simulink model "VCP_interface_STM32F429"  (R2022b)
settings: Solver=FixedStepDiscrete  StartTime=0.0  StopTime=inf  FixedStep=Ts  RelTol=1e-3
InitFcn:
  | datafields_per_usb_transfer = 16;
  | bytes_per_usb_transfer = 16*4;
  | Ts = 10e-3;
libraries: instrumentseriallib x3
settings Model: Creator=oliver.dieterle  LastModifiedBy=oliver.dieterle
settings SolverCC: AlgebraicLoopSolver=TrustRegion
settings DataIOCC: LimitDataPoints=on  SaveFormat=Array  ReturnWorkspaceOutputs=off
settings OptimizationCC: BlockReduction=off  BooleanDataType=off  LifeSpan=inf
settings DebuggingCC: SaveWithParameterizedLinksMsg=none  UnderspecifiedInitializationDetection=Classic  MergeDetectMultiDrivingBlocksExec=none  SignalResolutionControl=TryResolveAllWithWarning  UnconnectedInputMsg=warning  UnconnectedOutputMsg=warning  UnconnectedLineMsg=warning  SFUnexpectedBacktrackingDiag=warning  SFNoUnconditionalDefaultTransitionDiag=warning  SFExecutionAtInitializationDiag=none  SFMachineParentedDataDiag=warning  ArithmeticOperatorsInVariantConditions=warning
settings HardwareCC: ProdBitPerPointer=32  ProdBitPerSizeT=32  ProdBitPerPtrDiffT=32  ProdLargestAtomicFloat=None  ProdIntDivRoundTo=Undefined  ProdEndianess=Unspecified  ProdWordSize=32  ProdHWDeviceType=32-bit Generic  TargetUnknown=on
settings ModelReferenceCC: EnableRefExpFcnMdlSchedulingChecks=on  PropagateSignalLabelsOutOfModel=off
settings SFSimCC: SimUseLocalCustomCode=off  CustomCodeUndefinedFunction=UseInterfaceOnly
settings RTWCC: RTWUseLocalCustomCode=off
settings CodeAppCC: StateflowObjectComments=on
settings GRTTargetCC: TargetLangStandard=C89/C90 (ANSI)
settings ConfigComp: CovMetricSettings=dw  CovSaveCumulativeToWorkspaceVar=on  CovSaveSingleToWorkspaceVar=on  CovExternalEMLEnable=off  CovSFcnEnable=off

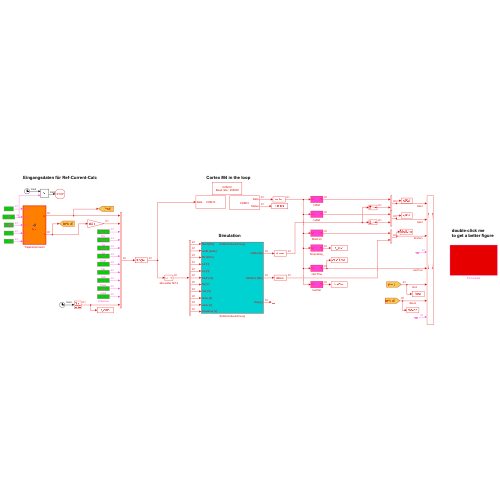
[thumbnail: Simulink's stored preview of the top-level diagram]
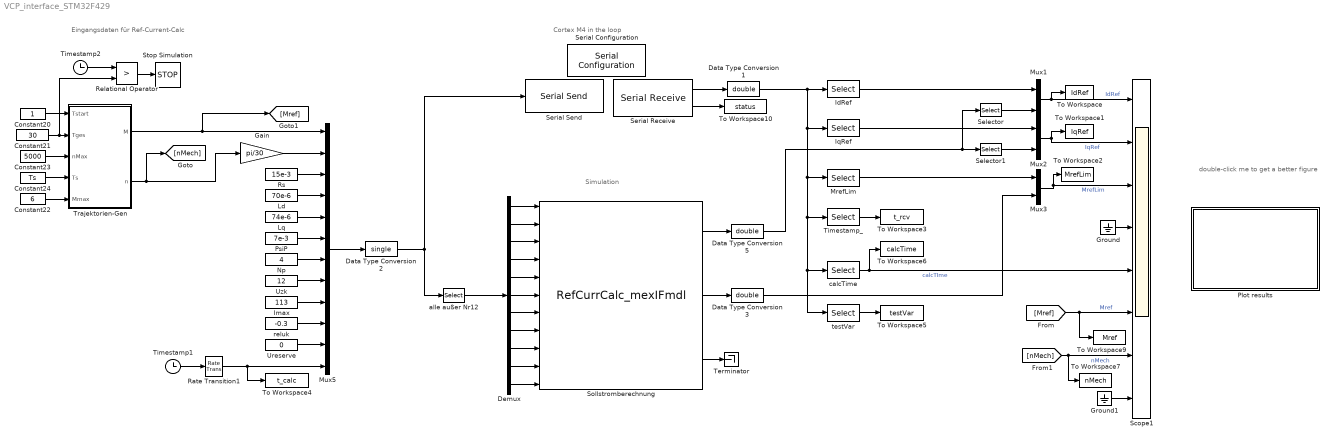
== system VCP_interface_STM32F429 ==
  note: Simulation
  note: Cortex M4 in the loop
  note: Eingangsdaten für Ref-Current-Calc
  note: double-click me
      | to get a better figure
  Constant20 : Constant
  Constant21 : Constant  Value=30
  Constant22 : Constant  Value=6
  Constant23 : Constant  Value=5000
  Constant24 : Constant  Value=Ts
  Data Type Conversion1 : DataTypeConversion  OutDataTypeStr=double  SaturateOnIntegerOverflow=off  RndMeth=Floor
  Data Type Conversion2 : DataTypeConversion  OutDataTypeStr=single  SaturateOnIntegerOverflow=off  RndMeth=Floor
  Data Type Conversion3 : DataTypeConversion  OutDataTypeStr=double  SaturateOnIntegerOverflow=off  RndMeth=Floor
  Data Type Conversion5 : DataTypeConversion  OutDataTypeStr=double  SaturateOnIntegerOverflow=off  RndMeth=Floor
  Demux : Demux  Outputs=11
  Gain : Gain  Gain=pi/30
  Ground : Ground
  Ground1 : Ground
  IdRef : Selector  InputPortWidth=datafields_per_usb_transfer  IndexOptions=Index vector (dialog)  Indices=1  OutputSizes=1
  Imax : Constant  Value=113
  IqRef : Selector  InputPortWidth=datafields_per_usb_transfer  IndexOptions=Index vector (dialog)  Indices=2  OutputSizes=1
  Ld : Constant  Value=70e-6
  Lq : Constant  Value=74e-6
  MrefLim : Selector  InputPortWidth=datafields_per_usb_transfer  IndexOptions=Index vector (dialog)  Indices=3  OutputSizes=1
  Mux1 : Mux  Inputs=2
  Mux2 : Mux  Inputs=2
  Mux3 : Mux  Inputs=2
  Mux5 : Mux  Inputs=12
  Np : Constant  Value=4
  Plot results : Subsystem
      settings: OpenFcn=plot_results;
  PsiP : Constant  Value=7e-3
  Rate Transition1 : RateTransition  OutPortSampleTime=Ts
  Relational Operator : RelationalOperator  Operator=>  OutDataTypeStr=boolean  RndMeth=Simplest  InputSameDT=off
  Rs : Constant  Value=15e-3
  Scope1 : Scope  NumInputPorts=8
  Selector : Selector  InputPortWidth=2  IndexOptions=Index vector (dialog)  Indices=1  OutputSizes=1
  Selector1 : Selector  InputPortWidth=2  IndexOptions=Index vector (dialog)  Indices=2  OutputSizes=1
  Serial Configuration : instrumentseriallib/Serial Configuration  Priority=-200000  PortSel=COM10  Port=COM10  ComPort=COM10  BaudRate=256000  DataBits=8  Parity=none  StopBits=1  ByteOrder=little-endian  FlowControl=none  Timeout=3  SimulateUsing=Interpreted execution  BlockInModel=on  aMode=1
  Serial Receive : instrumentseriallib/Serial Receive  PortSel=COM10  Port=COM10  ComPort=COM10  DataType=single  SaveDataType=uint8  ToggleHeader=on  Header="[ 72  69  65  68 ]"  ToggleTerminator=on  Terminator=<none>  CustomTerminator=[]  InputFormat=Column major  ToggleDataSize=on  DataSize="[16   1]"  EnableBlockingMode=off  ActionDataUnavailable=Output last received value  ActionWhenDataUnavailable=Output last received value  CustomValue=0  SampleTime=Ts  SimulateUsing=Interpreted execution  BlockInModel=on  aMode=1
  Serial Send : instrumentseriallib/Serial Send  PortSel=COM10  Port=COM10  ComPort=COM10  Header="[ 72  69  65  68 ]"  Terminator=<none>  CustomTerminator=[]  EnableBlockingMode=off  SimulateUsing=Interpreted execution  BlockInModel=on  aMode=1
  Sollstromberechnung : S-Function  FunctionName=RefCurrCalc_mexIFmdl  SFunctionModules='D:\Programming\CCode\Sollstromberechnung\Implementierung_v03\Test_in_Matlab\RefCurrentCalculation_main_Full'  SFunctionDeploymentMode=off  EnableBusSupport=off
      mask Display:
      | text(0.3,0.97,'Sollstromberechnung')
      | 
      | port_label('input', 1, 'Mref [Nm]')
      | port_label('input', 2, 'omEl [rad/s]')
      | port_label('input', 3, 'Rs [Ohm]')
      | port_label('input', 4, 'Ld [H]')
      | port_label('input', 5, 'Lq [H]')
      | port_label('input', 6, 'PsiP [Vs]')
      | port_label('input', 7, 'Np [1]')
      | port_label('input', 8, 'Uzk [V]')
      | port_label('input', 9, 'Imax [A]')
      | port_label('input', 10, 'reluk [V]')
      | port_label('input', 11, 'Ureserve [V]')
      | 
      | port_label('output', 1, 'IdqRef [A]')
      | port_label('output', 2, 'MrefLim [Nm]')
      | port_label('output', 3, 'diag [-]')
  Stop Simulation : Stop
  Terminator : Terminator
  Timestamp1 : Clock
  Timestamp2 : Clock
  Timestamp_ : Selector  InputPortWidth=datafields_per_usb_transfer  IndexOptions=Index vector (dialog)  Indices=4  OutputSizes=1
  To Workspace : ToWorkspace  VariableName=IdRef  SampleTime=Ts
  To Workspace1 : ToWorkspace  VariableName=IqRef  SampleTime=Ts
  To Workspace10 : ToWorkspace  VariableName=status  SaveFormat=Timeseries  SampleTime=Ts
  To Workspace2 : ToWorkspace  VariableName=MrefLim  SampleTime=Ts
  To Workspace3 : ToWorkspace  VariableName=t_rcv  SampleTime=Ts
  To Workspace4 : ToWorkspace  VariableName=t_calc  SampleTime=Ts
  To Workspace5 : ToWorkspace  VariableName=testVar  SampleTime=Ts
  To Workspace6 : ToWorkspace  VariableName=calcTime  SampleTime=Ts
  To Workspace7 : ToWorkspace  VariableName=nMech  SampleTime=Ts
  To Workspace9 : ToWorkspace  VariableName=Mref  SampleTime=Ts
  Trajektorien-Gen : MATLAB Function  TreatAsAtomicUnit=on  SystemSampleTime=Ts
  Ureserve : Constant  Value=0
  Uzk : Constant  Value=12
  alle außer Nr12 : Selector  InputPortWidth=12  IndexOptions=Index vector (dialog)  Indices=(1:11)  OutputSizes=1
  calcTime : Selector  InputPortWidth=datafields_per_usb_transfer  IndexOptions=Index vector (dialog)  Indices=5  OutputSizes=1
  reluk : Constant  Value=-0.3
  testVar : Selector  InputPortWidth=datafields_per_usb_transfer  IndexOptions=Index vector (dialog)  Indices=6  OutputSizes=1
  wires:
  Data Type Conversion2/1 -> Serial Send/1, alle außer Nr12/1
  Serial Receive/2 -> To Workspace10/1
  Serial Receive/1 -> Data Type Conversion1/1
  Mux1/1 -> To Workspace/1, Scope1/1  "IdRef"
  Mux2/1 -> Scope1/2, To Workspace1/1  "IqRef"
  Mux3/1 -> To Workspace2/1, Scope1/3  "MrefLim"
  IdRef/1 -> Mux1/1
  IqRef/1 -> Mux2/1
  MrefLim/1 -> Mux3/1
  Selector/1 -> Mux1/2
  Selector1/1 -> Mux2/2
  Timestamp_/1 -> To Workspace3/1
  calcTime/1 -> To Workspace6/1, Scope1/5  "calcTIme"
  Demux/2 -> Sollstromberechnung/2
  Demux/1 -> Sollstromberechnung/1
  Demux/4 -> Sollstromberechnung/4
  Demux/6 -> Sollstromberechnung/6
  Demux/7 -> Sollstromberechnung/7
  Demux/8 -> Sollstromberechnung/8
  Demux/9 -> Sollstromberechnung/9
  Demux/10 -> Sollstromberechnung/10
  Demux/5 -> Sollstromberechnung/5
  Demux/3 -> Sollstromberechnung/3
  Demux/11 -> Sollstromberechnung/11
  Trajektorien-Gen/1(M) -> [Mref], Mux5/1
  Rs/1 -> Mux5/3
  PsiP/1 -> Mux5/6
  Np/1 -> Mux5/7
  Uzk/1 -> Mux5/8
  Imax/1 -> Mux5/9
  reluk/1 -> Mux5/10
  Ureserve/1 -> Mux5/11
  Sollstromberechnung/1 -> Data Type Conversion5/1
  Sollstromberechnung/2 -> Data Type Conversion3/1
  Trajektorien-Gen/2(n) -> [nMech], Gain/1
  [Mref] -> To Workspace9/1, Scope1/6  "Mref"
  [nMech] -> To Workspace7/1, Scope1/7  "nMech"
  Timestamp1/1 -> Rate Transition1/1
  alle außer Nr12/1 -> Demux/1
  Data Type Conversion1/1 -> IdRef/1, IqRef/1, testVar/1, calcTime/1, Timestamp_/1, MrefLim/1
  Data Type Conversion3/1 -> Mux3/2
  Data Type Conversion5/1 -> Selector/1, Selector1/1
  Constant20/1 -> Trajektorien-Gen/1(Tstart)
  Constant24/1 -> Trajektorien-Gen/4(Ts)
  Constant23/1 -> Trajektorien-Gen/3(nMax)
  Constant22/1 -> Trajektorien-Gen/5(Mmax)
  Gain/1 -> Mux5/2
  Relational Operator/1 -> Stop Simulation/1
  Timestamp2/1 -> Relational Operator/1
  Mux5/1 -> Data Type Conversion2/1
  Rate Transition1/1 -> To Workspace4/1, Mux5/12
  Constant21/1 -> Relational Operator/2, Trajektorien-Gen/2(Tges)
  Lq/1 -> Mux5/5
  Ld/1 -> Mux5/4
  Ground/1 -> Scope1/4
  Sollstromberechnung/3 -> Terminator/1
  Ground1/1 -> Scope1/8
  testVar/1 -> To Workspace5/1

== system VCP_interface_STM32F429/Plot results ==

== matlab function VCP_interface_STM32F429/Trajektorien-Gen ==
  data: Tstart input; M output; Tges input; nMax input; Ts input; Mmax input; n output
function [M,n] = fcn(Tstart,Tges,nMax,Ts,Mmax)

persistent t

if(isempty(t)) t = 0; end

Tges = Tges/2;

t = t+Ts;
dn = nMax/Tges;


M = 0;
n = 0;

t_sin = t-Tstart;
    
if(t > Tstart+2*Tges)
    M = 0;
    n = 0;    
elseif(t > Tstart+2*Tges)
    M = Mmax*sin(2*pi*t_sin/(2*Tges));
    n = -dn*(t-(Tstart+2*Tges));
elseif(t > Tstart+Tges)
    M = Mmax*sin(2*pi*t_sin/(2*Tges));
    n = nMax - dn*(t-(Tstart+Tges));
elseif(t > Tstart)
    M = Mmax*sin(2*pi*t_sin/(2*Tges));
    n = dn*(t-Tstart);
end

end
